simulink model "CSVReadWriteSerial"  (R2017b)
settings: Solver=FixedStepDiscrete  StartTime=0.0  StopTime=10.0  FixedStep=1e-3  RelTol=1e-3
libraries: mbed_lib x5
settings Model: Creator=oh  LastModifiedBy=oh
settings OptimizationCC: DefaultParameterBehavior=Inlined  PassReuseOutputArgsAs=Individual arguments
settings DebuggingCC: ParameterTunabilityLossMsg=error
settings HardwareCC: ProdBitPerPointer=32  ProdBitPerSizeT=32  ProdBitPerPtrDiffT=32  ProdLargestAtomicInteger=Long  ProdLargestAtomicFloat=Double  ProdWordSize=32  ProdHWDeviceType=ARM Compatible->ARM Cortex
settings SFSimCC: MATLABDynamicMemAlloc=off
settings RTWCC: SystemTargetFile=mbed.tlc  TemplateMakefile=mbed.tmf  Description=MbedTarget (Embedded Target for Embedded Coder)  IncludeHyperlinkInReport=on  TargetLang=C++
settings CodeAppCC: ForceParamTrailComments=on  IgnoreCustomStorageClasses=off  OperatorAnnotations=on  SimulinkDataObjDesc=on  SFDataObjDesc=on  InsertBlockDesc=on
settings STFCustomTargetCC: TargetLibSuffix=.a  TargetLangStandard=C++03 (ISO)  MultiwordLength=256  GenerateSampleERTMain=on  CombineOutputUpdateFcns=on  ERTCustomFileBanners=on  SupportContinuousTime=off  SupportNonInlinedSFcns=off  RemoveResetFunc=on  MATLABClassNameForMDSCustomization=Simulink.SoftwareTarget.ERTCustomization  ModelStepFunctionPrototypeControlCompliant=on  GRTInterface=off  SystemTargetFile=mbed.tlc
settings ERTTargetCC: TargetLangStandard=C++03 (ISO)  GenerateSampleERTMain=on  ParMdlRefBuildCompliant=off  CompOptLevelCompliant=off  ConcurrentExecutionCompliant=off  CPPClassGenCompliant=off  UseToolchainInfoCompliant=off  InlinedParameterPlacement=NonHierarchical  ERTCustomFileTemplate=mbed_file_process.tlc

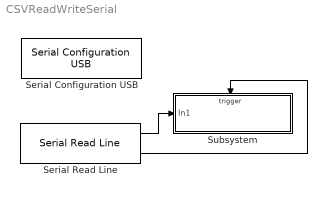
== system CSVReadWriteSerial ==
  Serial Configuration USB : mbed_lib/Serial/UART/Serial Configuration USB  Priority=0  BaudRate=9600
      settings: SourceProductName=Mbed Target
  Serial Read Line : mbed_lib/Serial/UART/Serial Read Line  SerialPort=USB  NumDataPort=off  NewDataPort=on  BufferSize=100  SampleTime=-1
      settings: SourceProductName=Mbed Target
  Subsystem : Subsystem
  wires:
  Serial Read Line/1 -> Subsystem/1(In1)
  Serial Read Line/2 -> Subsystem/Trigger

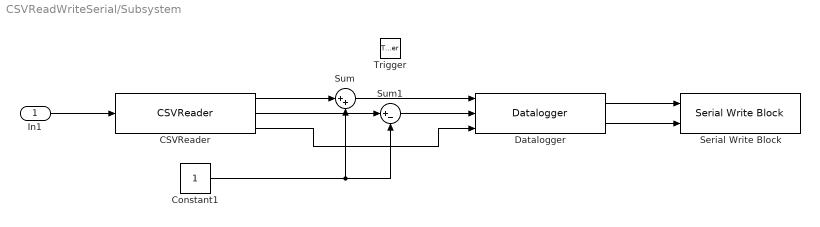
== system CSVReadWriteSerial/Subsystem ==
  In1 : Inport  OutDataTypeStr=uint8
  Trigger : TriggerPort  VariantControl=Variant  PortDimensions=1
  CSVReader : mbed_lib/Utilities/CSVReader  TypeOutputPorts={ 'uint8' 1 'int16' 1 'single' 1 }  TypeOfOutputs={'1*uint8' '1*int16' '1*single'}  BufferSize=0  SampleTime=-1
      settings: SourceProductName=Mbed Target
  Constant1 : Constant  OutDataTypeStr=Inherit: Inherit via back propagation
  Datalogger : mbed_lib/Utilities/Datalogger  TypeInputPorts={ 'uint8' 1 'int16' 1 'single' 1 }  TypeOfInputs={'1*uint8' '1*int16' '1*single'}  BufferSize=100  errEn=off  SampleTime=-1
      settings: SourceProductName=Mbed Target
  Serial Write Block : mbed_lib/Serial/UART/Serial Write Block  SerialPort=USB  numData=on  SampleTime=-1
      settings: SourceProductName=Mbed Target
  Sum : Sum  Inputs=|++  OutDataTypeStr=uint8
  Sum1 : Sum  Inputs=|+-  OutDataTypeStr=int16
  wires:
  CSVReader/3 -> Datalogger/3
  Datalogger/1 -> Serial Write Block/1
  Datalogger/2 -> Serial Write Block/2
  In1/1 -> CSVReader/1
  CSVReader/1 -> Sum/1
  Sum1/1 -> Datalogger/2
  Sum/1 -> Datalogger/1
  CSVReader/2 -> Sum1/1
  Constant1/1 -> Sum/2, Sum1/2
